simulink model "MSIP_Speed_Control_abc1a_84"  (R2025a)
settings: Solver=FixedStepAuto  StartTime=0.0  StopTime=150  FixedStep=1e-4  MaxStep=1e-3  RelTol=1e-3
model workspace (MAT data in the model file):
  Freq = 60
values from neighbouring files (symbols this model uses):
  b_MS = 1e-3    (= 0.001)    [data_MSIP_julio2025.m]
  beta_d_MS = pd_MS    (= 40)    [data_MSIP_julio2025.m]
  gamq = 2*J_MS*Lq_MS/(3*np_MS*lambda_MS)    (= 0.00452625826005)    [data_MSIP_julio2025.m]
  J_MS = 1e-1    (= 0.1)    [data_MSIP_julio2025.m]
  lambda_MS = 67.09e-2    (= 0.6709)    [data_MSIP_julio2025.m]
  Ld_MS = 22.1e-3    (= 0.0221)    [data_MSIP_julio2025.m]
  Lq_MS = 91.1e-3    (= 0.0911)    [data_MSIP_julio2025.m]
  np_MS = 2    [data_MSIP_julio2025.m]
  Rs_MS = 6.51e-1    (= 0.651)    [data_MSIP_julio2025.m]
undefined symbols (not defined in the file or in its folder): plecs
libraries: plecslib_extras2 x3, spsRMSLib x2, spsPLL3phLib x1, nesl_utility x1, spsTHDLib x1
(part 2 of 2)

== matlab function MSIP_Speed_Control_abc1a_84/Subsystem/Theta_Deseada1 ==
  data: t input; ys output
function ys = theta_deseada2(t)
    
t1 = 50;   %  " initial and final instants of rest-to-rest
t2 = 60;

delt = t2-t1;
tdif = abs(t-t1) ;

% " initial and final values 
z1in = 0;
z1f  = (-100) + 1800*2*pi/60;

%z1f  = dta0;

z1dif = z1f-z1in;

tau=(tdif/delt);
tau2=tau*tau;
tau3=tau*tau2;
tau4=tau*tau3;
tau5=tau*tau4;
tau6=tau*tau5;
tau7=tau*tau6;
tau8=tau*tau7;
tau9=tau*tau8;

r1=12870;
r2=91520;
r3=288288;
r4=524160;
r5=600600;
r6=443520;
r7=205920;
r8=54912;
r9=6435;

z1st1 = z1in;
fr    = r1-r2*tau+r3*tau2-r4*tau3+r5*tau4-r6*tau5+r7*tau6-r8*tau7+r9*tau8;
z1stt = z1in+z1dif*tau8*fr;
z1st2 = z1f;


    if t<t1
         ys     = z1st1; 
    elseif t<t2
         ys     = z1stt; 
    else
         ys     = z1st2; 
    end

== matlab function MSIP_Speed_Control_abc1a_84/3 Nm/TL1 ==
  data: t input; T_load output
function T_load = Tload(t)
    
t1 = 30;   %  " initial and final instants of rest-to-rest
t2 = 40;

delt = t2-t1;
tdif = abs(t-t1) ;

% " initial and final values 
z1in = 0;
z1f  = 30;

%z1f  = dta0;

z1dif = z1f-z1in;

tau=(tdif/delt);
tau2=tau*tau;
tau3=tau*tau2;
tau4=tau*tau3;
tau5=tau*tau4;
tau6=tau*tau5;
tau7=tau*tau6;
tau8=tau*tau7;
tau9=tau*tau8;

r1=12870;
r2=91520;
r3=288288;
r4=524160;
r5=600600;
r6=443520;
r7=205920;
r8=54912;
r9=6435;

z1st1 = z1in;
fr    = r1-r2*tau+r3*tau2-r4*tau3+r5*tau4-r6*tau5+r7*tau6-r8*tau7+r9*tau8;
z1stt = z1in+z1dif*tau8*fr;
z1st2 = z1f;


    if t<t1
         T_load     = z1st1; 
    elseif t<t2
         T_load     = z1stt; 
    else
         T_load     = z1st2; 
    end

== matlab function MSIP_Speed_Control_abc1a_84/Subsystem/Theta_Deseada2 ==
  data: t input; ys output
function ys = theta_deseada3(t)
    
t1 = 105;   %  " initial and final instants of rest-to-rest
t2 = 110;

delt = t2-t1;
tdif = abs(t-t1) ;

% " initial and final values 
z1in = 0;
z1f  = -1600*2*pi/60;

%z1f  = dta0;

z1dif = z1f-z1in;

tau=(tdif/delt);
tau2=tau*tau;
tau3=tau*tau2;
tau4=tau*tau3;
tau5=tau*tau4;
tau6=tau*tau5;
tau7=tau*tau6;
tau8=tau*tau7;
tau9=tau*tau8;

r1=12870;
r2=91520;
r3=288288;
r4=524160;
r5=600600;
r6=443520;
r7=205920;
r8=54912;
r9=6435;

z1st1 = z1in;
fr    = r1-r2*tau+r3*tau2-r4*tau3+r5*tau4-r6*tau5+r7*tau6-r8*tau7+r9*tau8;
z1stt = z1in+z1dif*tau8*fr;
z1st2 = z1f;


    if t<t1
         ys     = z1st1; 
    elseif t<t2
         ys     = z1stt; 
    else
         ys     = z1st2; 
    end

== matlab function MSIP_Speed_Control_abc1a_84/b)VSC_84/PULSES_7L/MATLAB Function ==
  data: u input; s1 output; s2 output; s3 output; s4 output; s5 output; s6 output; s7 output; s8 output
function [s1,s2,s3,s4,s5,s6,s7,s8]= fcn(u)
    if u>13*0.0748 %pi/42=0.0748
        s1=1;s2=1;s3=0;s4=0;s5=0;s6=0;s7=1;s8=1;        
    elseif u>12*0.0748
        s1=0;s2=1;s3=1;s4=0;s5=0;s6=0;s7=1;s8=1;
    elseif u>11*0.0748
        s1=1;s2=1;s3=0;s4=0;s5=0;s6=1;s7=1;s8=0;
    elseif u>10*0.0748
        s1=0;s2=1;s3=1;s4=0;s5=0;s6=1;s7=1;s8=0;        
    elseif u>9*0.0748
        s1=0;s2=0;s3=1;s4=1;s5=0;s6=1;s7=1;s8=0;
    elseif u>8*0.0748
        s1=0;s2=1;s3=1;s4=0;s5=1;s6=1;s7=0;s8=0;
    elseif u>7*0.0748
        s1=0;s2=0;s3=1;s4=1;s5=1;s6=1;s7=0;s8=0;
    elseif u>6*0.0748
        s1=0;s2=0;s3=1;s4=1;s5=1;s6=1;s7=0;s8=0;
    elseif u>5*0.0748
        s1=0;s2=1;s3=1;s4=0;s5=1;s6=1;s7=0;s8=0;
    elseif u>4*0.0748
        s1=0;s2=0;s3=1;s4=1;s5=0;s6=1;s7=1;s8=0;
    elseif u>3*0.0748
        s1=0;s2=1;s3=1;s4=0;s5=0;s6=1;s7=1;s8=0;        
    elseif u>2*0.0748
        s1=1;s2=1;s3=0;s4=0;s5=0;s6=1;s7=1;s8=0;
    elseif u>(0.0748)
        s1=0;s2=1;s3=1;s4=0;s5=0;s6=0;s7=1;s8=1;
    elseif u>0
        s1=1;s2=1;s3=0;s4=0;s5=0;s6=0;s7=1;s8=1;
    else
        s1=0;s2=0;s3=0;s4=0;s5=0;s6=0;s7=0;s8=0;
    
end

== matlab function MSIP_Speed_Control_abc1a_84/b)VSC_84/PULSES_YD/MATLAB Function ==
  data: u input; s1 output; s2 output; s3 output; s4 output; s5 output; s6 output
function [s1,s2,s3,s4,s5,s6]= fcn(u)
    if  u>5*1.0472 %pi/3=1.0472
        s1=0;s2=0;s3=0;s4=1;s5=1;s6=1;
    elseif u>4*1.0472
        s1=0;s2=0;s3=1;s4=1;s5=1;s6=0;
    elseif u>pi
        s1=0;s2=1;s3=1;s4=1;s5=0;s6=0;        
    elseif u>2*1.0472
        s1=1;s2=1;s3=1;s4=0;s5=0;s6=0;
    elseif u>(1.0472)
        s1=1;s2=1;s3=0;s4=0;s5=0;s6=1;
    elseif u>0
        s1=1;s2=0;s3=0;s4=0;s5=1;s6=1;
    else
        s1=0;s2=0;s3=0;s4=0;s5=0;s6=0;
    
end

== matlab function MSIP_Speed_Control_abc1a_84/Subsystem/Theta_Deseada ==
  data: t input; ys output
function ys = theta_deseada(t)
    
t1 = 5;   %  " initial and final instants of rest-to-rest
t2 = 20;

delt = t2-t1;
tdif = abs(t-t1) ;

% " initial and final values 
z1in = 0;
z1f  = 100;


z1dif = z1f-z1in;

tau=(tdif/delt);
tau2=tau*tau;
tau3=tau*tau2;
tau4=tau*tau3;
tau5=tau*tau4;
tau6=tau*tau5;
tau7=tau*tau6;
tau8=tau*tau7;
tau9=tau*tau8;

r1=12870;
r2=91520;
r3=288288;
r4=524160;
r5=600600;
r6=443520;
r7=205920;
r8=54912;
r9=6435;

z1st1 = z1in;
fr    = r1-r2*tau+r3*tau2-r4*tau3+r5*tau4-r6*tau5+r7*tau6-r8*tau7+r9*tau8;
z1stt = z1in+z1dif*tau8*fr;
z1st2 = z1f;


    if t<t1
         ys     = z1st1; 
    elseif t<t2
         ys     = z1stt; 
    else
         ys     = z1st2; 
    end

== matlab function MSIP_Speed_Control_abc1a_84/Module ==
  data: Phi_V input; angle output; Phi_I input
function angle = fcn(Phi_V,Phi_I)
   % angle = mod(Phi_V - Phi_I , 2*pi) ;
    %angle = mod(Phi_V - Phi_I , 2*pi) ;
    if (Phi_V-Phi_I<0) angle=Phi_V-Phi_I+2*pi; else angle=Phi_V-Phi_I;
end

== matlab function MSIP_Speed_Control_abc1a_84/PLL1/Module ==
  data: u input; y output
function y = fcn(u)
if (and(u(1)==0,u(2)==0))
    y=1;
else
    y = sqrt(u(1)*u(1)+u(2)*u(2));
end

== matlab function MSIP_Speed_Control_abc1a_84/PLL2/Module ==
  data: u input; y output
function y = fcn(u)
if (and(u(1)==0,u(2)==0))
    y=1;
else
    y = sqrt(u(1)*u(1)+u(2)*u(2));
end

== matlab function MSIP_Speed_Control_abc1a_84/b)VSC_84/Module ==
  data: u input; y output
function y = fcn(u)
max=21440000;
min=0.1;
%if abs(u(1)) < 0.00010 && abs(u(2)) < 0.00010 && abs(u(3)) < 0.00010
%    u(:) = 0;
%end
module=sqrt(u(1)*u(1)+u(2)*u(2)+u(3)*u(3));
if(module>max)
    y=max;
elseif(module<min)
    y=min;
else
    y=module;
end
%y=sqrt(u(1)*u(1)+u(2)*u(2)+u(3)*u(3));
